simulink model "simulation"  (R2024b)
settings: Solver=FixedStepAuto  StartTime=0.0  StopTime=10  FixedStep=0.005  RelTol=1e-3
undefined symbols (not defined in the file): drawaircraft, Earth, force_moment, fractalcoef, MAV, Payload, sample_time, SIM, WGS84
libraries: uavmavlinklib x8, simulink x2, robotcorelib x1, sensorgpslib x1, mspsensorlib x1, aerolibatmos2 x1, sharedtransform x1, aerolibtransform2 x1
settings Model: Creator=SJ  LastModifiedBy=SJ

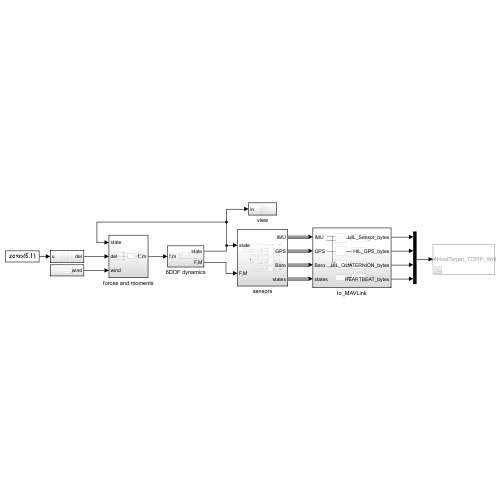
[thumbnail: Simulink's stored preview of the top-level diagram]
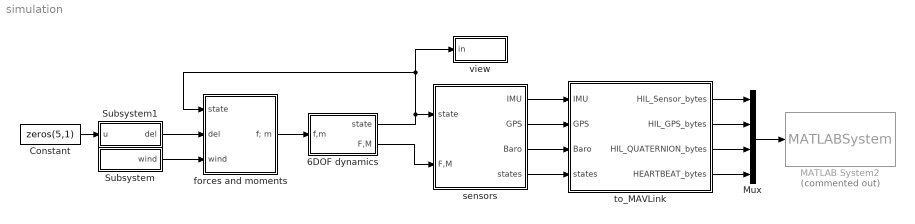
== system simulation ==
  6DOF dynamics : Subsystem
  Constant : Constant  Value=zeros(5,1)
  MATLAB System2 : MATLABSystem  Commented=on  System=px4HostTarget_TCPIP_Write
      mask Type: px4HostTarget_TCPIP_Write
      mask Display: disp('px4HostTarget_TCPIP_Write');
  Mux : Mux
  Subsystem : Subsystem
  Subsystem1 : Subsystem
  forces and moments : Subsystem
  sensors : Subsystem
  to_MAVLink : Subsystem
  view : Subsystem
  wires:
  Subsystem/1(wind) -> forces and moments/3(wind)
  forces and moments/1(f; m) -> 6DOF dynamics/1(f,m)
  Subsystem1/1(del) -> forces and moments/2(del)
  Constant/1 -> Subsystem1/1(u)
  6DOF dynamics/1(state) -> forces and moments/1(state), view/1(in), sensors/1(state)
  6DOF dynamics/2(F,M) -> sensors/2(F,M)
  sensors/1(IMU) -> to_MAVLink/1(IMU)
  sensors/3(Baro) -> to_MAVLink/3(Baro)
  sensors/2(GPS) -> to_MAVLink/2(GPS)
  sensors/4(states) -> to_MAVLink/4(states)
  Mux/1 -> MATLAB System2/1
  to_MAVLink/1(HIL_Sensor_bytes) -> Mux/1
  to_MAVLink/2(HIL_GPS_bytes) -> Mux/2
  to_MAVLink/3(HIL_QUATERNION_bytes) -> Mux/3
  to_MAVLink/4(HEARTBEAT_bytes) -> Mux/4

== system simulation/6DOF dynamics ==
  f,m : Inport
  S-Function : S-Function  FunctionName=UAVdynamics  Parameters=MAV  SFunctionDeploymentMode=off  EnableBusSupport=off
  state : Outport
  F,M : Outport  Port=2
  wires:
  f,m/1 -> F,M/1, S-Function/1
  S-Function/1 -> state/1  "state"

== system simulation/Subsystem ==
  Constant16 : Constant  Value=[SIM.wind.wn_s; SIM.wind.we_s; SIM.wind.wd_s]
  Constant17 : Constant  Value=[0; 0; 0]
  Mux1 : Mux  Inputs=2
  wind : Outport
  wires:
  Constant17/1 -> Mux1/2
  Mux1/1 -> wind/1  "wind"
  Constant16/1 -> Mux1/1

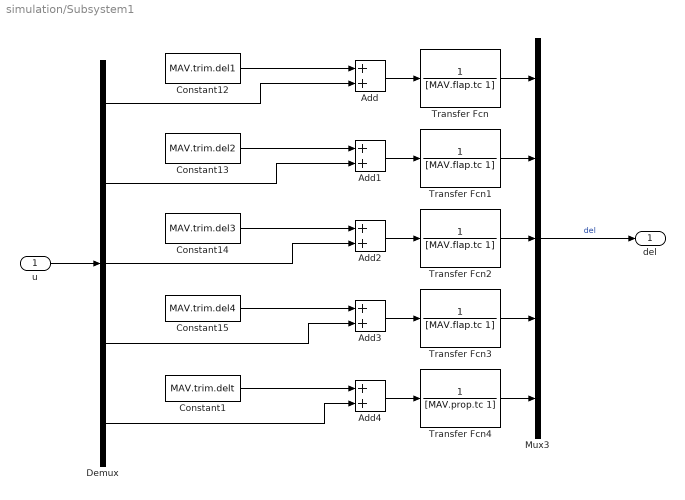
== system simulation/Subsystem1 ==
  u : Inport
  Add{,1..4} (5 alike) : Sum
  Constant1 : Constant  Value=MAV.trim.delt
  Constant12 : Constant  Value=MAV.trim.del1
  Constant13 : Constant  Value=MAV.trim.del2
  Constant14 : Constant  Value=MAV.trim.del3
  Constant15 : Constant  Value=MAV.trim.del4
  Demux : Demux  Outputs=5
  Mux3 : Mux  Inputs=5
  Transfer Fcn{,1..3} (4 alike) : TransferFcn  Denominator=[MAV.flap.tc 1]
  Transfer Fcn4 : TransferFcn  Denominator=[MAV.prop.tc 1]
  del : Outport
  wires:
  Mux3/1 -> del/1  "del"
  Constant15/1 -> Add3/1
  Constant13/1 -> Add1/1
  Constant12/1 -> Add/1
  Constant14/1 -> Add2/1
  Constant1/1 -> Add4/1
  Demux/1 -> Add/2
  Demux/2 -> Add1/2
  Demux/3 -> Add2/2
  Demux/4 -> Add3/2
  Demux/5 -> Add4/2
  u/1 -> Demux/1
  Add/1 -> Transfer Fcn/1
  Add1/1 -> Transfer Fcn1/1
  Add2/1 -> Transfer Fcn2/1
  Add3/1 -> Transfer Fcn3/1
  Add4/1 -> Transfer Fcn4/1
  Transfer Fcn/1 -> Mux3/1
  Transfer Fcn4/1 -> Mux3/5
  Transfer Fcn1/1 -> Mux3/2
  Transfer Fcn3/1 -> Mux3/4
  Transfer Fcn2/1 -> Mux3/3

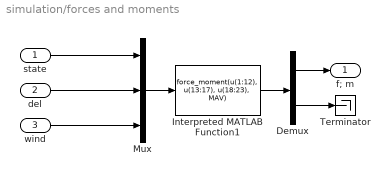
== system simulation/forces and moments ==
  state : Inport
  del : Inport  Port=2
  wind : Inport  Port=3
  Demux : Demux  Outputs=[6,3]
  Interpreted MATLAB Function1 : MATLABFcn  MATLABFcn=force_moment(u(1:12), u(13:17), u(18:23), MAV)  OutputDimensions=9
  Mux : Mux  Inputs=3
  Terminator : Terminator
  f; m : Outport
  wires:
  Mux/1 -> Interpreted MATLAB Function1/1
  state/1 -> Mux/1
  del/1 -> Mux/2
  wind/1 -> Mux/3
  Interpreted MATLAB Function1/1 -> Demux/1
  Demux/1 -> f; m/1
  Demux/2 -> Terminator/1

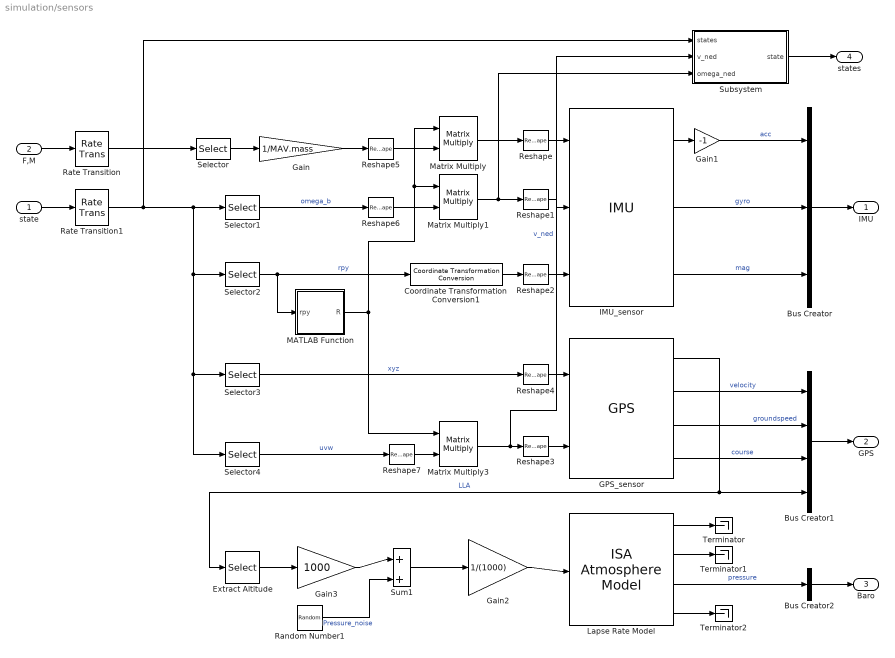
== system simulation/sensors ==
  state : Inport
  F,M : Inport  Port=2
  Bus Creator : BusCreator  Inputs=3
  Bus Creator1 : BusCreator  Inputs=4
  Bus Creator2 : BusCreator  Inputs=1
  Coordinate Transformation Conversion1 : robotcorelib/Coordinate Transformation Conversion  InputRepresentation=Euler Angles  InputEulerSequence=ZYX  ShowTrVecInputPort=on  OutputRepresentation=Quaternion  OutputEulerSequence=ZYX  ShowTrVecOutputPort=on  SimulateUsing=Interpreted execution
  Extract Altitude : Selector  InputPortWidth=3  IndexOptions=Index vector (dialog)  Indices=[3]  OutputSizes=1
  GPS_sensor : sensorgpslib/GPS  DispRefFrame=NED  PositionInputFormat=Local  ReferenceLocation=[ 0, 0, 0 ]  HorizontalPositionAccuracy=1.6  VerticalPositionAccuracy=3  VelocityAccuracy=0.1  DecayFactor=0.999  SeedDouble=67  SimulateUsing=Interpreted execution
      settings: LibrarySourceBlock=uavsimlib/GPS
  Gain : Gain  Gain=1/MAV.mass
  Gain1 : Gain  Gain=-1
  Gain2 : Gain  Gain=1/(1000)
  Gain3 : Gain  Gain=1000
  IMU_sensor : mspsensorlib/IMU  DispRefFrame=NED  TemperaturePort=off  Temperature=25  MagneticFieldPort=off  MagneticFieldNED=[ 27.5550, -2.4169, -16.0849 ]  MagneticFieldENU=[ -2.4169, 27.5550, 16.0849 ]  SeedDouble=67  SimulateUsing=Interpreted execution  AccelParamsMeasurementRange=Inf  AccelParamsResolution=0  AccelParamsConstantBias=[ 0, 0, 0 ]  AccelParamsAxesMisalignment=[ 100, 0, 0; 0, 100, 0; 0, 0, 100 ]  AccelParamsNoiseDensity=[ 0, 0, 0 ]  AccelParamsBiasInstability=[ 0, 0, 0 ]  AccelParamsBiasInstabilityNumerator=fractalcoef().Numerator  AccelParamsBiasInstabilityDenominator=fractalcoef().Denominator  AccelParamsRandomWalk=[ 0, 0, 0 ]  AccelParamsNoiseType=double-sided  AccelParamsTemperatureBias=[ 0, 0, 0 ]  AccelParamsTemperatureScaleFactor=[ 0, 0, 0 ]  GyroParamsMeasurementRange=Inf  GyroParamsResolution=0  GyroParamsConstantBias=[ 0, 0, 0 ]  GyroParamsAxesMisalignment=[ 100, 0, 0; 0, 100, 0; 0, 0, 100 ]  GyroParamsAccelerationBias=[ 0, 0, 0 ]  GyroParamsNoiseDensity=[ 0, 0, 0 ]  GyroParamsBiasInstability=[ 0, 0, 0 ]  GyroParamsBiasInstabilityNumerator=fractalcoef().Numerator  GyroParamsBiasInstabilityDenominator=fractalcoef().Denominator  GyroParamsRandomWalk=[ 0, 0, 0 ]  GyroParamsNoiseType=double-sided  GyroParamsTemperatureBias=[ 0, 0, 0 ]  GyroParamsTemperatureScaleFactor=[ 0, 0, 0 ]  MagParamsMeasurementRange=Inf  MagParamsResolution=0  MagParamsConstantBias=[ 0, 0, 0 ]  MagParamsAxesMisalignment=[ 100, 0, 0; 0, 100, 0; 0, 0, 100 ]  MagParamsNoiseDensity=[ 0, 0, 0 ]  MagParamsBiasInstability=[ 0, 0, 0 ]  MagParamsBiasInstabilityNumerator=fractalcoef().Numerator  MagParamsBiasInstabilityDenominator=fractalcoef().Denominator  MagParamsRandomWalk=[ 0, 0, 0 ]  MagParamsNoiseType=double-sided  MagParamsTemperatureBias=[ 0, 0, 0 ]  MagParamsTemperatureScaleFactor=[ 0, 0, 0 ]
  Lapse Rate Model : aerolibatmos2/ISA Atmosphere Model  useExtended=off  action=Warning  custom=on  viscosityOut=off  g=9.80665  gamma=1.4  R=287.0531  L=0.0065  h_trop=11000  h_strat=20000  rho0=1.225  P0=101325  T0=288.15  h0=0  S=110.4  Tref=273.15  muref=1.716e-5
  MATLAB Function : MATLAB Function  TreatAsAtomicUnit=on
  Matrix Multiply : Product  Multiplication=Matrix(*)
  Matrix Multiply1 : Product  Multiplication=Matrix(*)
  Matrix Multiply3 : Product  Multiplication=Matrix(*)
  Random Number1 : RandomNumber  Variance=10000  Seed=10  SampleTime=sample_time
  Rate Transition : RateTransition  OutPortSampleTime=0.01
  Rate Transition1 : RateTransition  OutPortSampleTime=0.01
  Reshape{,1..4} (5 alike) : Reshape  OutputDimensionality=Row vector (2-D)
  Reshape5 : Reshape  OutputDimensionality=Column vector (2-D)
  Reshape6 : Reshape  OutputDimensionality=Column vector (2-D)
  Reshape7 : Reshape  OutputDimensionality=Column vector (2-D)
  Selector : Selector  InputPortWidth=6  IndexOptions=Index vector (dialog)  Indices=[1:3]  OutputSizes=1
  Selector1 : Selector  InputPortWidth=12  IndexOptions=Index vector (dialog)  Indices=[10:12]  OutputSizes=1
  Selector2 : Selector  InputPortWidth=12  IndexOptions=Index vector (dialog)  Indices=[7:9]  OutputSizes=1
  Selector3 : Selector  InputPortWidth=12  IndexOptions=Index vector (dialog)  Indices=[1:3]  OutputSizes=1
  Selector4 : Selector  InputPortWidth=12  IndexOptions=Index vector (dialog)  Indices=[4:6]  OutputSizes=1
  Subsystem : Subsystem
  Sum1 : Sum  Inputs=|++
  Terminator : Terminator
  Terminator1 : Terminator
  Terminator2 : Terminator
  IMU : Outport
  GPS : Outport  Port=2
  Baro : Outport  Port=3
  states : Outport  Port=4
  wires:
  Reshape/1 -> IMU_sensor/1
  Selector2/1 -> Coordinate Transformation Conversion1/1, MATLAB Function/1(rpy)  "rpy"
  Reshape1/1 -> IMU_sensor/2
  Coordinate Transformation Conversion1/1 -> Reshape2/1
  Reshape2/1 -> IMU_sensor/3
  IMU_sensor/1 -> Gain1/1
  IMU_sensor/2 -> Bus Creator/2  "gyro"
  IMU_sensor/3 -> Bus Creator/3  "mag"
  F,M/1 -> Rate Transition/1
  Matrix Multiply/1 -> Reshape/1
  MATLAB Function/1(R) -> Matrix Multiply/1, Matrix Multiply1/1, Matrix Multiply3/1
  Matrix Multiply1/1 -> Subsystem/3(omega_ned), Reshape1/1
  Selector1/1 -> Reshape6/1  "omega_b"
  Gain/1 -> Reshape5/1
  Selector/1 -> Gain/1
  state/1 -> Rate Transition1/1
  Selector3/1 -> Reshape4/1  "xyz"
  Matrix Multiply3/1 -> Subsystem/2(v_ned), Reshape3/1  "v_ned"
  Selector4/1 -> Reshape7/1  "uvw"
  Gain1/1 -> Bus Creator/1  "acc"
  Reshape3/1 -> GPS_sensor/2
  Reshape4/1 -> GPS_sensor/1
  GPS_sensor/2 -> Bus Creator1/1  "velocity"
  GPS_sensor/3 -> Bus Creator1/2  "groundspeed"
  GPS_sensor/4 -> Bus Creator1/3  "course"
  Reshape6/1 -> Matrix Multiply1/2
  Reshape7/1 -> Matrix Multiply3/2
  Reshape5/1 -> Matrix Multiply/2
  Random Number1/1 -> Sum1/2  "Pressure_noise"
  Extract Altitude/1 -> Gain3/1
  Lapse Rate Model/3 -> Bus Creator2/1  "pressure"
  Gain2/1 -> Lapse Rate Model/1
  Lapse Rate Model/2 -> Terminator1/1
  Gain3/1 -> Sum1/1
  Lapse Rate Model/4 -> Terminator2/1
  Sum1/1 -> Gain2/1
  Lapse Rate Model/1 -> Terminator/1
  GPS_sensor/1 -> Extract Altitude/1, Bus Creator1/4  "LLA"
  Rate Transition/1 -> Selector/1
  Rate Transition1/1 -> Subsystem/1(states), Selector4/1, Selector3/1, Selector2/1, Selector1/1
  Bus Creator/1 -> IMU/1
  Bus Creator1/1 -> GPS/1
  Bus Creator2/1 -> Baro/1
  Subsystem/1(state) -> states/1

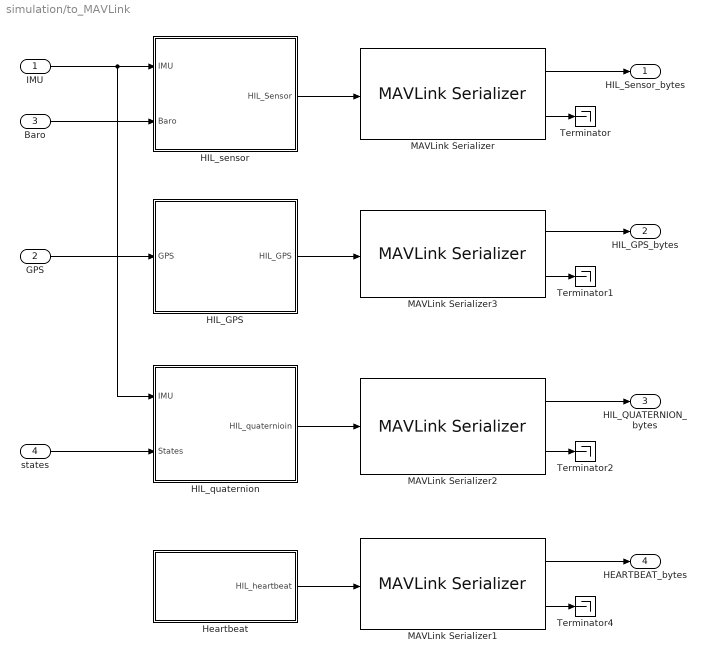
== system simulation/to_MAVLink ==
  IMU : Inport
  GPS : Inport  Port=2
  Baro : Inport  Port=3
  states : Inport  Port=4
  HIL_GPS : Subsystem
  HIL_quaternion : Subsystem
  HIL_sensor : Subsystem
  Heartbeat : Subsystem
  MAVLink Serializer : uavmavlinklib/MAVLink Serializer  dialectSource=Select from standard MAVLink dialects  dialect=common.xml  dialectCustom=common.xml  version=2  messageType=HIL_SENSOR
  MAVLink Serializer1 : uavmavlinklib/MAVLink Serializer  dialectSource=Select from standard MAVLink dialects  dialect=common.xml  dialectCustom=common.xml  version=2  messageType=HEARTBEAT
  MAVLink Serializer2 : uavmavlinklib/MAVLink Serializer  dialectSource=Select from standard MAVLink dialects  dialect=common.xml  dialectCustom=common.xml  version=2  messageType=HIL_STATE_QUATERNION
  MAVLink Serializer3 : uavmavlinklib/MAVLink Serializer  dialectSource=Select from standard MAVLink dialects  dialect=common.xml  dialectCustom=common.xml  version=2  messageType=HIL_GPS
  Terminator{,1..2,4} (4 alike) : Terminator
  HIL_Sensor_bytes : Outport
  HIL_GPS_bytes : Outport  Port=2
  HIL_QUATERNION_bytes : Outport  Port=3
  HEARTBEAT_bytes : Outport  Port=4
  wires:
  IMU/1 -> HIL_quaternion/1(IMU), HIL_sensor/1(IMU)
  Baro/1 -> HIL_sensor/2(Baro)
  HIL_sensor/1(HIL_Sensor) -> MAVLink Serializer/1
  MAVLink Serializer/1 -> HIL_Sensor_bytes/1
  MAVLink Serializer/2 -> Terminator/1
  HIL_GPS/1(HIL_GPS) -> MAVLink Serializer3/1
  GPS/1 -> HIL_GPS/1(GPS)
  MAVLink Serializer3/1 -> HIL_GPS_bytes/1
  MAVLink Serializer3/2 -> Terminator1/1
  states/1 -> HIL_quaternion/2(States)
  MAVLink Serializer2/2 -> Terminator2/1
  MAVLink Serializer2/1 -> HIL_QUATERNION_bytes/1
  HIL_quaternion/1(HIL_quaternioin) -> MAVLink Serializer2/1
  MAVLink Serializer1/1 -> HEARTBEAT_bytes/1
  MAVLink Serializer1/2 -> Terminator4/1
  Heartbeat/1(HIL_heartbeat) -> MAVLink Serializer1/1

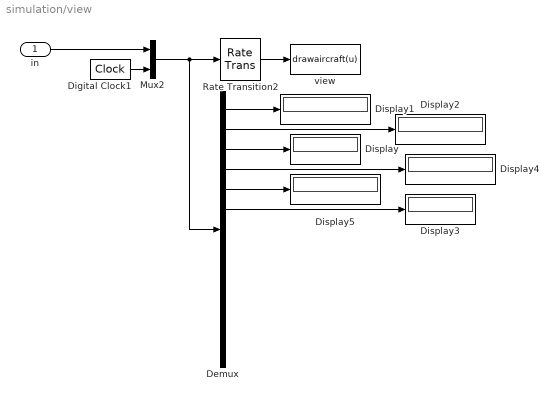
== system simulation/view ==
  in : Inport
  Demux : Demux  Outputs=13
  Digital Clock1 : DigitalClock  SampleTime=0.005
  Display{,1..5} (6 alike) : Display
  Mux2 : Mux  Inputs=2
  Rate Transition2 : RateTransition  OutPortSampleTime=0.1
  view : MATLABFcn  MATLABFcn=drawaircraft(u)  OutputDimensions=0
  wires:
  Rate Transition2/1 -> view/1
  Digital Clock1/1 -> Mux2/2
  Mux2/1 -> Demux/1, Rate Transition2/1
  in/1 -> Mux2/1
  Demux/3 -> Display/1
  Demux/1 -> Display1/1
  Demux/2 -> Display2/1
  Demux/4 -> Display4/1
  Demux/5 -> Display5/1
  Demux/6 -> Display3/1

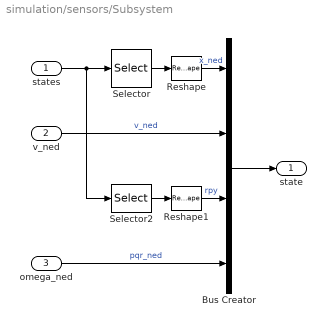
== system simulation/sensors/Subsystem ==
  states : Inport
  v_ned : Inport  Port=2
  omega_ned : Inport  Port=3
  Bus Creator : BusCreator  Inputs=4
  Reshape : Reshape  OutputDimensionality=Column vector (2-D)
  Reshape1 : Reshape  OutputDimensionality=Column vector (2-D)
  Selector : Selector  InputPortWidth=12  IndexOptions=Index vector (dialog)  Indices=[1:3]  OutputSizes=1
  Selector2 : Selector  InputPortWidth=12  IndexOptions=Index vector (dialog)  Indices=[7:9]  OutputSizes=1
  state : Outport
  wires:
  states/1 -> Selector2/1, Selector/1
  Selector/1 -> Reshape/1
  v_ned/1 -> Bus Creator/2  "v_ned"
  Selector2/1 -> Reshape1/1
  omega_ned/1 -> Bus Creator/4  "pqr_ned"
  Bus Creator/1 -> state/1
  Reshape/1 -> Bus Creator/1  "x_ned"
  Reshape1/1 -> Bus Creator/3  "rpy"

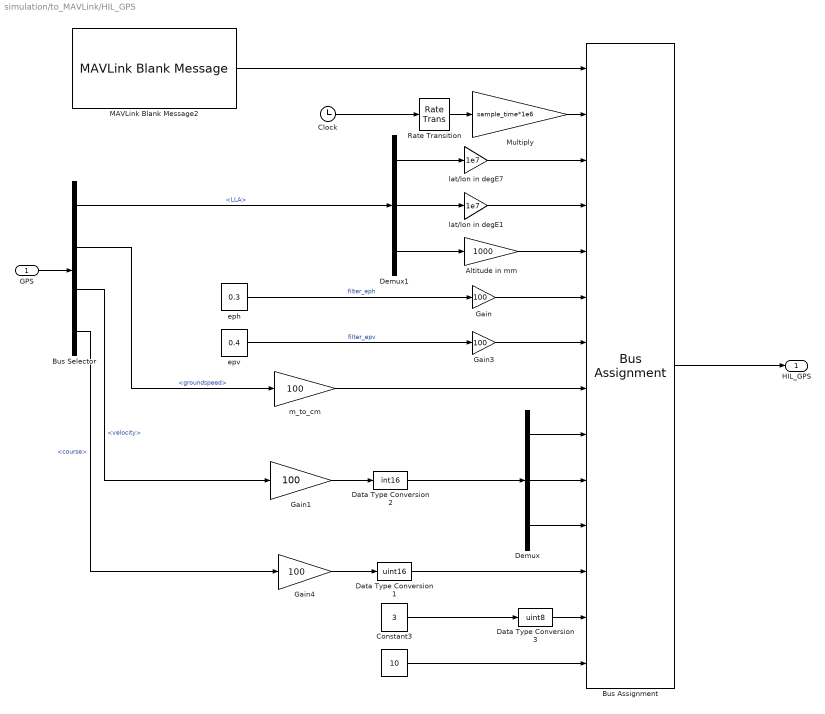
== system simulation/to_MAVLink/HIL_GPS ==
  GPS : Inport
  " " : Constant  Value=10  OutDataTypeStr=Inherit: Inherit via back propagation  SampleTime=-1
  Altitude in mm : Gain  Gain=1000  OutDataTypeStr=Inherit: Inherit via back propagation
  Bus Assignment : BusAssignment  AssignedSignals=Payload.time_usec,Payload.lat,Payload.lon,Payload.alt,Payload.eph,Payload.epv,Payload.vel,Payload.vn,Payload.ve,Payload.vd,Payload.cog,Payload.fix_type,Payload.satellites_visible
  Bus Selector : BusSelector  OutputSignals=LLA,groundspeed,velocity,course
  Clock : Clock
  Constant3 : Constant  Value=3  OutDataTypeStr=Inherit: Inherit via back propagation  SampleTime=-1
  Data Type Conversion1 : DataTypeConversion  OutDataTypeStr=uint16  SaturateOnIntegerOverflow=off  RndMeth=Floor
  Data Type Conversion2 : DataTypeConversion  OutDataTypeStr=int16  SaturateOnIntegerOverflow=off  RndMeth=Floor
  Data Type Conversion3 : DataTypeConversion  OutDataTypeStr=uint8  SaturateOnIntegerOverflow=off  RndMeth=Floor
  Demux : Demux  Outputs=3
  Demux1 : Demux  Outputs=3
  Gain : Gain  Gain=100  OutDataTypeStr=Inherit: Inherit via back propagation
  Gain1 : Gain  Gain=100
  Gain3 : Gain  Gain=100  OutDataTypeStr=Inherit: Inherit via back propagation
  Gain4 : Gain  Gain=100
  MAVLink Blank Message2 : uavmavlinklib/MAVLink Blank Message  dialectSource=Select from standard MAVLink dialects  dialect=common.xml  dialectCustom=common.xml  version=2  messageType=HIL_GPS  SystemID=2  ComponentID=51  SampleTime=sample_time
  Multiply : Gain  Gain=sample_time*1e6  OutDataTypeStr=Inherit: Inherit via back propagation
  Rate Transition : RateTransition
  eph : Constant  Value=0.3  SampleTime=-1
  epv : Constant  Value=0.4  SampleTime=-1
  lat/lon in degE1 : Gain  Gain=1e7  OutDataTypeStr=Inherit: Inherit via back propagation
  lat/lon in degE7 : Gain  Gain=1e7  OutDataTypeStr=Inherit: Inherit via back propagation
  m_to_cm : Gain  Gain=100  OutDataTypeStr=uint16
  HIL_GPS : Outport
  wires:
  m_to_cm/1 -> Bus Assignment/8
  lat/lon in degE7/1 -> Bus Assignment/3
  Demux1/1 -> lat/lon in degE7/1
  Demux/3 -> Bus Assignment/11
  MAVLink Blank Message2/1 -> Bus Assignment/1
  Gain1/1 -> Data Type Conversion2/1
  Demux1/3 -> Altitude in mm/1
  Demux1/2 -> lat/lon in degE1/1
  Demux/1 -> Bus Assignment/9
  lat/lon in degE1/1 -> Bus Assignment/4
  Altitude in mm/1 -> Bus Assignment/5
  Data Type Conversion2/1 -> Demux/1
  Demux/2 -> Bus Assignment/10
  Bus Assignment/1 -> HIL_GPS/1
  " "/1 -> Bus Assignment/14
  Gain/1 -> Bus Assignment/6
  Gain3/1 -> Bus Assignment/7
  Bus Selector/2 -> m_to_cm/1  "<groundspeed>"
  Bus Selector/3 -> Gain1/1  "<velocity>"
  Bus Selector/4 -> Gain4/1  "<course>"
  Data Type Conversion1/1 -> Bus Assignment/12
  eph/1 -> Gain/1  "filter_eph"
  epv/1 -> Gain3/1  "filter_epv"
  Data Type Conversion3/1 -> Bus Assignment/13
  Gain4/1 -> Data Type Conversion1/1
  Constant3/1 -> Data Type Conversion3/1
  Clock/1 -> Rate Transition/1
  Rate Transition/1 -> Multiply/1
  Multiply/1 -> Bus Assignment/2
  GPS/1 -> Bus Selector/1
  Bus Selector/1 -> Demux1/1  "<LLA>"

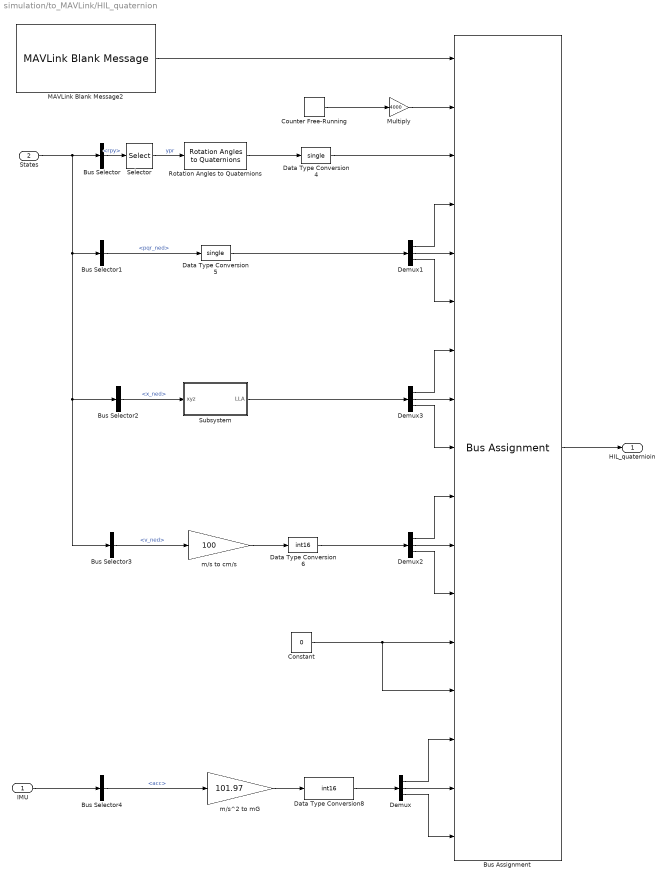
== system simulation/to_MAVLink/HIL_quaternion ==
  IMU : Inport
  States : Inport  Port=2
  Bus Assignment : BusAssignment  AssignedSignals=Payload.time_usec,Payload.attitude_quaternion,Payload.rollspeed,Payload.pitchspeed,Payload.yawspeed,Payload.lat,Payload.lon,Payload.alt,Payload.vx,Payload.vy,Payload.vz,Payload.ind_airspeed,Payload.true_airspeed,Payload.xacc,Payload.yacc,Payload.zacc
  Bus Selector : BusSelector  OutputSignals=rpy
  Bus Selector1 : BusSelector  OutputSignals=pqr_ned
  Bus Selector2 : BusSelector  OutputSignals=x_ned
  Bus Selector3 : BusSelector  OutputSignals=v_ned
  Bus Selector4 : BusSelector  OutputSignals=acc
  Constant : Constant  Value=0  OutDataTypeStr=Inherit: Inherit via back propagation
  Counter Free-Running : simulink/Sources/Counter Free-Running  NumBits=64  tsamp=-1
  Data Type Conversion4 : DataTypeConversion  OutDataTypeStr=single  SaturateOnIntegerOverflow=off  RndMeth=Floor
  Data Type Conversion5 : DataTypeConversion  OutDataTypeStr=single  SaturateOnIntegerOverflow=off  RndMeth=Floor
  Data Type Conversion6 : DataTypeConversion  OutDataTypeStr=int16  SaturateOnIntegerOverflow=off  RndMeth=Floor
  Data Type Conversion8 : DataTypeConversion  OutDataTypeStr=int16  SaturateOnIntegerOverflow=off  RndMeth=Floor
  Demux{,1..3} (4 alike) : Demux  Outputs=3
  MAVLink Blank Message2 : uavmavlinklib/MAVLink Blank Message  dialectSource=Select from standard MAVLink dialects  dialect=common.xml  dialectCustom=common.xml  version=2  messageType=HIL_STATE_QUATERNION  SystemID=2  ComponentID=51  SampleTime=sample_time
  Multiply : Gain  Gain=4000  OutDataTypeStr=Inherit: Inherit via back propagation
  Rotation Angles to Quaternions : sharedtransform/Rotation Angles to Quaternions  rotationOrder=ZYX  aMode=aMode
  Selector : Selector  InputPortWidth=3  IndexOptions=Index vector (dialog)  Indices=[3 2 1]  OutputSizes=1
  Subsystem : Subsystem
  m/s to cm/s : Gain  Gain=100
  m/s^2 to mG : Gain  Gain=101.97
  HIL_quaternioin : Outport
  wires:
  Multiply/1 -> Bus Assignment/2
  Data Type Conversion8/1 -> Demux/1
  Data Type Conversion6/1 -> Demux2/1
  Demux2/1 -> Bus Assignment/10
  Demux3/2 -> Bus Assignment/8
  Demux1/3 -> Bus Assignment/6
  Demux/1 -> Bus Assignment/15
  Subsystem/1(LLA) -> Demux3/1
  MAVLink Blank Message2/1 -> Bus Assignment/1
  m/s to cm/s/1 -> Data Type Conversion6/1
  Bus Selector1/1 -> Data Type Conversion5/1  "<pqr_ned>"
  Data Type Conversion4/1 -> Bus Assignment/3
  Demux2/3 -> Bus Assignment/12
  Data Type Conversion5/1 -> Demux1/1
  Demux/2 -> Bus Assignment/16
  Demux3/3 -> Bus Assignment/9
  Demux/3 -> Bus Assignment/17
  Rotation Angles to Quaternions/1 -> Data Type Conversion4/1
  Demux3/1 -> Bus Assignment/7
  m/s^2 to mG/1 -> Data Type Conversion8/1
  States/1 -> Bus Selector/1, Bus Selector1/1, Bus Selector3/1, Bus Selector2/1
  Constant/1 -> Bus Assignment/14, Bus Assignment/13
  Demux2/2 -> Bus Assignment/11
  Counter Free-Running/1 -> Multiply/1
  Demux1/1 -> Bus Assignment/4
  Demux1/2 -> Bus Assignment/5
  IMU/1 -> Bus Selector4/1
  Bus Assignment/1 -> HIL_quaternioin/1
  Selector/1 -> Rotation Angles to Quaternions/1  "ypr"
  Bus Selector2/1 -> Subsystem/1(xyz)  "<x_ned>"
  Bus Selector/1 -> Selector/1  "<rpy>"
  Bus Selector3/1 -> m/s to cm/s/1  "<v_ned>"
  Bus Selector4/1 -> m/s^2 to mG/1  "<acc>"

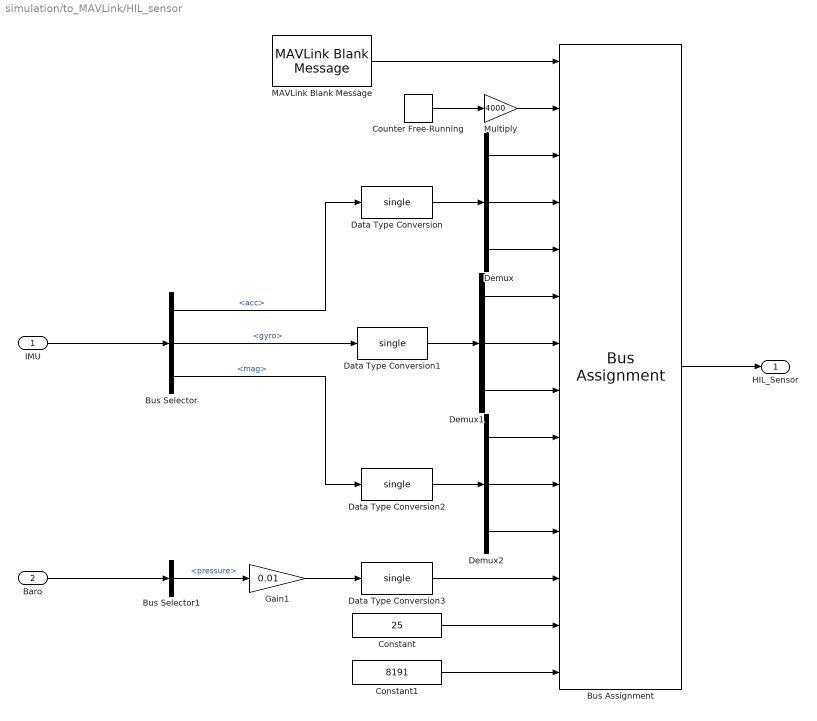
== system simulation/to_MAVLink/HIL_sensor ==
  IMU : Inport
  Baro : Inport  Port=2
  Bus Assignment : BusAssignment  AssignedSignals=Payload.time_usec,Payload.xacc,Payload.yacc,Payload.zacc,Payload.xgyro,Payload.ygyro,Payload.zgyro,Payload.xmag,Payload.ymag,Payload.zmag,Payload.abs_pressure,Payload.temperature,Payload.fields_updated
  Bus Selector : BusSelector  OutputSignals=acc,gyro,mag
  Bus Selector1 : BusSelector  OutputSignals=pressure
  Constant : Constant  Value=25  OutDataTypeStr=single  SampleTime=sample_time
  Constant1 : Constant  Value=8191  OutDataTypeStr=uint32  SampleTime=sample_time
  Counter Free-Running : simulink/Sources/Counter Free-Running  NumBits=64  tsamp=sample_time
  Data Type Conversion{,1..3} (4 alike) : DataTypeConversion  OutDataTypeStr=single  SaturateOnIntegerOverflow=off  RndMeth=Floor
  Demux : Demux  Outputs=3
  Demux1 : Demux  Outputs=3
  Demux2 : Demux  Outputs=3
  Gain1 : Gain  Gain=0.01
  MAVLink Blank Message : uavmavlinklib/MAVLink Blank Message  dialectSource=Select from standard MAVLink dialects  dialect=common.xml  dialectCustom=common.xml  version=2  messageType=HIL_SENSOR  SystemID=2  ComponentID=51  SampleTime=sample_time
  Multiply : Gain  Gain=4000  OutDataTypeStr=Inherit: Inherit via back propagation
  HIL_Sensor : Outport
  wires:
  IMU/1 -> Bus Selector/1
  MAVLink Blank Message/1 -> Bus Assignment/1
  Multiply/1 -> Bus Assignment/2
  Demux/3 -> Bus Assignment/5
  Demux/1 -> Bus Assignment/3
  Demux/2 -> Bus Assignment/4
  Demux1/1 -> Bus Assignment/6
  Demux1/2 -> Bus Assignment/7
  Demux1/3 -> Bus Assignment/8
  Demux2/1 -> Bus Assignment/9
  Demux2/2 -> Bus Assignment/10
  Demux2/3 -> Bus Assignment/11
  Bus Selector/1 -> Data Type Conversion/1  "<acc>"
  Bus Selector/2 -> Data Type Conversion1/1  "<gyro>"
  Bus Selector/3 -> Data Type Conversion2/1  "<mag>"
  Data Type Conversion/1 -> Demux/1
  Data Type Conversion1/1 -> Demux1/1
  Data Type Conversion2/1 -> Demux2/1
  Baro/1 -> Bus Selector1/1
  Bus Selector1/1 -> Gain1/1  "<pressure>"
  Data Type Conversion3/1 -> Bus Assignment/12
  Constant/1 -> Bus Assignment/13
  Constant1/1 -> Bus Assignment/14
  Gain1/1 -> Data Type Conversion3/1
  Bus Assignment/1 -> HIL_Sensor/1
  Counter Free-Running/1 -> Multiply/1

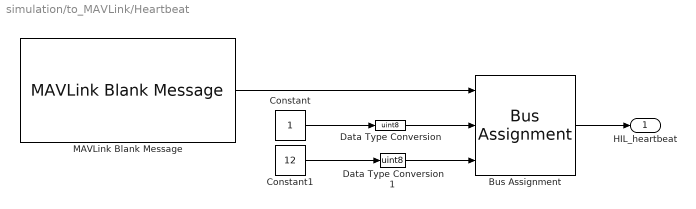
== system simulation/to_MAVLink/Heartbeat ==
  Bus Assignment : BusAssignment  AssignedSignals=Payload.autopilot,Payload.type
  Constant : Constant  SampleTime=sample_time
  Constant1 : Constant  Value=12  SampleTime=sample_time
  Data Type Conversion : DataTypeConversion  OutDataTypeStr=uint8  SaturateOnIntegerOverflow=off  RndMeth=Floor
  Data Type Conversion1 : DataTypeConversion  OutDataTypeStr=uint8  SaturateOnIntegerOverflow=off  RndMeth=Floor
  MAVLink Blank Message : uavmavlinklib/MAVLink Blank Message  dialectSource=Select from standard MAVLink dialects  dialect=common.xml  dialectCustom=common.xml  version=2  messageType=HEARTBEAT  SystemID=2  ComponentID=51  SampleTime=sample_time
  HIL_heartbeat : Outport
  wires:
  Constant/1 -> Data Type Conversion/1
  Data Type Conversion1/1 -> Bus Assignment/3
  Data Type Conversion/1 -> Bus Assignment/2
  Constant1/1 -> Data Type Conversion1/1
  MAVLink Blank Message/1 -> Bus Assignment/1
  Bus Assignment/1 -> HIL_heartbeat/1

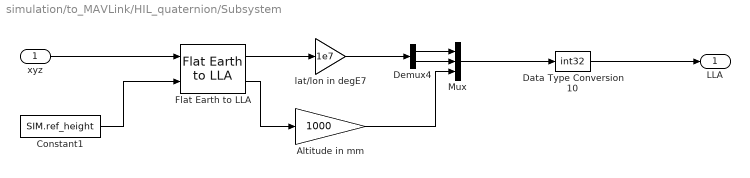
== system simulation/to_MAVLink/HIL_quaternion/Subsystem ==
  xyz : Inport
  Altitude in mm : Gain  Gain=1000
  Constant1 : Constant  Value=SIM.ref_height  OutDataTypeStr=Inherit: Inherit via back propagation
  Data Type Conversion10 : DataTypeConversion  OutDataTypeStr=int32  SaturateOnIntegerOverflow=off  RndMeth=Floor
  Demux4 : Demux  Outputs=2
  Flat Earth to LLA : aerolibtransform2/Flat Earth to LLA  units=Metric (MKS)  ptype=Earth (WGS84)  F=1/298.257223563  R=6378137  refPosPort=off  LL0=[0 10]  psi=0
  Mux : Mux  Inputs=3
  lat/lon in degE7 : Gain  Gain=1e7
  LLA : Outport
  wires:
  Flat Earth to LLA/2 -> Altitude in mm/1
  Demux4/1 -> Mux/1
  Constant1/1 -> Flat Earth to LLA/2
  Altitude in mm/1 -> Mux/3
  Mux/1 -> Data Type Conversion10/1
  Data Type Conversion10/1 -> LLA/1
  xyz/1 -> Flat Earth to LLA/1
  lat/lon in degE7/1 -> Demux4/1
  Flat Earth to LLA/1 -> lat/lon in degE7/1
  Demux4/2 -> Mux/2

== matlab function simulation/sensors/MATLAB Function ==
  data: rpy input; R output
function R = rotate_b2i(rpy)
    phi = rpy(1); theta = rpy(2); psi = rpy(3);
    R_psi = [cos(psi), sin(psi), 0;
            -sin(psi), cos(psi), 0
            0, 0, 1];
    R_theta = [cos(theta), 0, -sin(theta);
                0 , 1, 0;
                sin(theta), 0, cos(theta)];
    R_phi = [1, 0, 0;
             0, cos(phi), sin(phi);
             0, -sin(phi), cos(phi)];
    R = R_phi * R_theta * R_psi;
    R = R';
end
